simulink model "Duffing_Oszillator_Simulation"  (R2018b)
settings: Solver=VariableStepAuto  StartTime=0.0  StopTime=30  RelTol=1e-3
values from neighbouring files (symbols this model uses):
  a_alpha = 0.95    [Duffing_Oszillator_Parameter.m]
  a_delta = 0.95    [Duffing_Oszillator_Parameter.m]
  alpha_w = 1    [Duffing_Oszillator_Parameter.m]
  beta_w = -1    [Duffing_Oszillator_Parameter.m]
  delta_ksi = (0.3-(-0.3))/(r-1)    (= 0.03)    [Duffing_Oszillator_Parameter.m]
  delta_w = 0.2    [Duffing_Oszillator_Parameter.m]
  eta_alpha = 7*10^(-2)    (= 0.07)    [Duffing_Oszillator_Parameter.m]
  eta_delta = 1.5*10^(-3)    (= 0.0015)    [Duffing_Oszillator_Parameter.m]
  gamma_w = 10    [Duffing_Oszillator_Parameter.m]
  h = 0.001    [Duffing_Oszillator_Parameter.m]
  ksi = linspace(-0.3,0.3,r)    [Duffing_Oszillator_Parameter.m]
  l1 = 10    [Duffing_Oszillator_Parameter.m]
  l2 = 1.75    [Duffing_Oszillator_Parameter.m]
  omega_0 = 6    [Duffing_Oszillator_Parameter.m]
  r = 21    [Duffing_Oszillator_Parameter.m]
  sigma_norm = 0.3    [Duffing_Oszillator_Parameter.m]
undefined symbols (not defined in the file or in its folder): a_theta, DiscIntNeverNeededParam, eta_theta
settings Model: Creator=LENOVO  LastModifiedBy=LENOVO

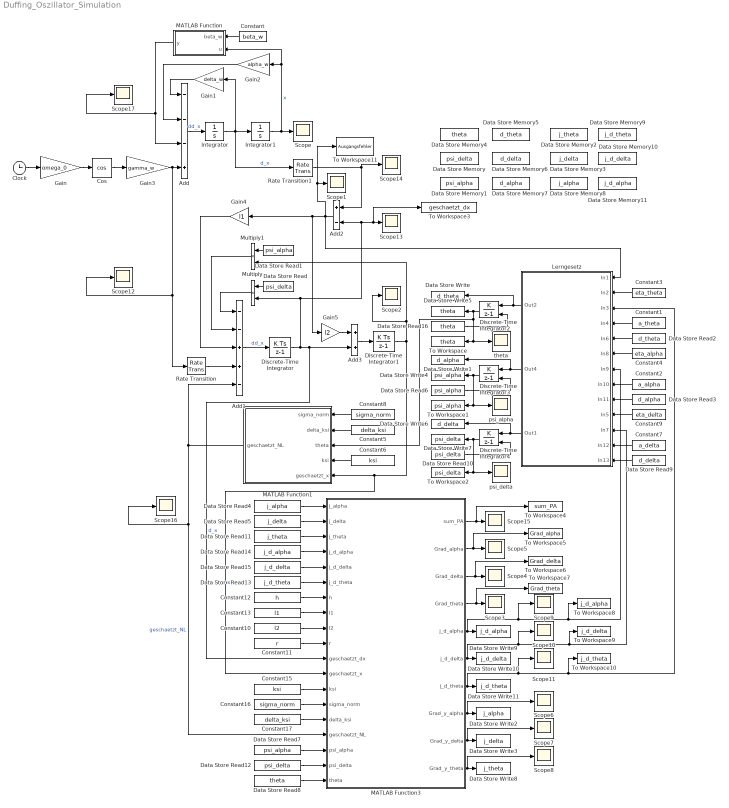
== system Duffing_Oszillator_Simulation ==
  Add : Sum  Inputs=---+
  Add1 : Sum  Inputs=--++-
  Add2 : Sum  Inputs=+-
  Add3 : Sum
  Clock : Clock
  Constant : Constant  Value=beta_w
  Constant1 : Constant  Value=a_theta
  Constant10 : Constant  Value=l2
  Constant11 : Constant  Value=r
  Constant12 : Constant  Value=h
  Constant13 : Constant  Value=l1
  Constant15 : Constant  Value=ksi
  Constant16 : Constant  Value=sigma_norm
  Constant17 : Constant  Value=delta_ksi
  Constant2 : Constant  Value=a_alpha
  Constant3 : Constant  Value=eta_theta
  Constant4 : Constant  Value=eta_alpha
  Constant5 : Constant  Value=delta_ksi
  Constant6 : Constant  Value=ksi
  Constant7 : Constant  Value=a_delta
  Constant8 : Constant  Value=sigma_norm
  Constant9 : Constant  Value=eta_delta
  Cos : Trigonometry  Operator=cos
  Data Store Memory : DataStoreMemory  DataStoreName=psi_delta  ReadBeforeWriteMsg=warning  WriteAfterWriteMsg=warning  WriteAfterReadMsg=warning  InitialValue=0.3  ShowAdditionalParam=off
  Data Store Memory1 : DataStoreMemory  DataStoreName=psi_alpha  ReadBeforeWriteMsg=warning  WriteAfterWriteMsg=warning  WriteAfterReadMsg=warning  InitialValue=1.4  ShowAdditionalParam=off
  Data Store Memory10 : DataStoreMemory  DataStoreName=j_d_delta  ReadBeforeWriteMsg=warning  WriteAfterWriteMsg=warning  WriteAfterReadMsg=warning  ShowAdditionalParam=off
  Data Store Memory11 : DataStoreMemory  DataStoreName=j_d_alpha  ReadBeforeWriteMsg=warning  WriteAfterWriteMsg=warning  WriteAfterReadMsg=warning  ShowAdditionalParam=off
  Data Store Memory2 : DataStoreMemory  DataStoreName=j_theta  ReadBeforeWriteMsg=warning  WriteAfterWriteMsg=warning  WriteAfterReadMsg=warning  InitialValue=zeros(1,r)  ShowAdditionalParam=off
  Data Store Memory3 : DataStoreMemory  DataStoreName=j_delta  ReadBeforeWriteMsg=warning  WriteAfterWriteMsg=warning  WriteAfterReadMsg=warning  ShowAdditionalParam=off
  Data Store Memory4 : DataStoreMemory  DataStoreName=theta  ReadBeforeWriteMsg=warning  WriteAfterWriteMsg=warning  WriteAfterReadMsg=warning  InitialValue=zeros(1,r)  ShowAdditionalParam=off
  Data Store Memory5 : DataStoreMemory  DataStoreName=d_theta  ReadBeforeWriteMsg=warning  WriteAfterWriteMsg=warning  WriteAfterReadMsg=warning  InitialValue=zeros(1,r)  ShowAdditionalParam=off
  Data Store Memory6 : DataStoreMemory  DataStoreName=d_delta  ReadBeforeWriteMsg=warning  WriteAfterWriteMsg=warning  WriteAfterReadMsg=warning  ShowAdditionalParam=off
  Data Store Memory7 : DataStoreMemory  DataStoreName=d_alpha  ReadBeforeWriteMsg=warning  WriteAfterWriteMsg=warning  WriteAfterReadMsg=warning  ShowAdditionalParam=off
  Data Store Memory8 : DataStoreMemory  DataStoreName=j_alpha  ReadBeforeWriteMsg=warning  WriteAfterWriteMsg=warning  WriteAfterReadMsg=warning  ShowAdditionalParam=off
  Data Store Memory9 : DataStoreMemory  DataStoreName=j_d_theta  ReadBeforeWriteMsg=warning  WriteAfterWriteMsg=warning  WriteAfterReadMsg=warning  InitialValue=zeros(1,r)  ShowAdditionalParam=off
  Data Store Read : DataStoreRead  DataStoreName=psi_delta
  Data Store Read1 : DataStoreRead  DataStoreName=psi_alpha
  Data Store Read10 : DataStoreRead  DataStoreName=psi_delta
  Data Store Read11 : DataStoreRead  DataStoreName=j_theta
  Data Store Read12 : DataStoreRead  DataStoreName=psi_delta
  Data Store Read13 : DataStoreRead  DataStoreName=j_d_theta
  Data Store Read14 : DataStoreRead  DataStoreName=j_d_alpha
  Data Store Read15 : DataStoreRead  DataStoreName=j_d_delta
  Data Store Read16 : DataStoreRead  DataStoreName=theta
  Data Store Read2 : DataStoreRead  DataStoreName=d_theta
  Data Store Read3 : DataStoreRead  DataStoreName=d_alpha
  Data Store Read4 : DataStoreRead  DataStoreName=j_alpha
  Data Store Read5 : DataStoreRead  DataStoreName=j_delta
  Data Store Read6 : DataStoreRead  DataStoreName=psi_alpha
  Data Store Read7 : DataStoreRead  DataStoreName=psi_alpha
  Data Store Read8 : DataStoreRead  DataStoreName=theta
  Data Store Read9 : DataStoreRead  DataStoreName=d_delta
  Data Store Write : DataStoreWrite  DataStoreName=d_theta
  Data Store Write1 : DataStoreWrite  DataStoreName=d_alpha
  Data Store Write10 : DataStoreWrite  DataStoreName=j_d_delta
  Data Store Write11 : DataStoreWrite  DataStoreName=j_d_theta
  Data Store Write2 : DataStoreWrite  DataStoreName=j_alpha
  Data Store Write3 : DataStoreWrite  DataStoreName=j_delta
  Data Store Write4 : DataStoreWrite  DataStoreName=psi_alpha
  Data Store Write5 : DataStoreWrite  DataStoreName=theta
  Data Store Write6 : DataStoreWrite  DataStoreName=d_delta
  Data Store Write7 : DataStoreWrite  DataStoreName=psi_delta
  Data Store Write8 : DataStoreWrite  DataStoreName=j_theta
  Data Store Write9 : DataStoreWrite  DataStoreName=j_d_alpha
  Discrete-Time Integrator : DiscreteIntegrator  SampleTime=-1  ICPrevOutput=DiscIntNeverNeededParam  ICPrevScaledInput=DiscIntNeverNeededParam
  Discrete-Time Integrator1 : DiscreteIntegrator  InitialCondition=-0.3  SampleTime=-1  ICPrevOutput=DiscIntNeverNeededParam  ICPrevScaledInput=DiscIntNeverNeededParam
  Discrete-Time Integrator2 : DiscreteIntegrator  IntegratorMethod=Accumulation: Forward Euler  gainval=1  InitialConditionSource=external  SampleTime=-1  ICPrevOutput=DiscIntNeverNeededParam  ICPrevScaledInput=DiscIntNeverNeededParam
  Discrete-Time Integrator3 : DiscreteIntegrator  IntegratorMethod=Accumulation: Forward Euler  gainval=1  InitialConditionSource=external  SampleTime=-1  ICPrevOutput=DiscIntNeverNeededParam  ICPrevScaledInput=DiscIntNeverNeededParam
  Discrete-Time Integrator4 : DiscreteIntegrator  IntegratorMethod=Accumulation: Forward Euler  gainval=1  InitialConditionSource=external  SampleTime=-1  ICPrevOutput=DiscIntNeverNeededParam  ICPrevScaledInput=DiscIntNeverNeededParam
  Gain : Gain  Gain=omega_0
  Gain1 : Gain  Gain=delta_w
  Gain2 : Gain  Gain=alpha_w
  Gain3 : Gain  Gain=gamma_w
  Gain4 : Gain  Gain=l1
  Gain5 : Gain  Gain=l2
  Integrator : Integrator
  Integrator1 : Integrator  InitialCondition=-0.3
  Lerngesetz : Subsystem
  MATLAB Function : MATLAB Function  TreatAsAtomicUnit=on
  MATLAB Function1 : MATLAB Function  TreatAsAtomicUnit=on
  MATLAB Function3 : MATLAB Function  TreatAsAtomicUnit=on
  Multiply : Product
  Multiply1 : Product
  Rate Transition : RateTransition  OutPortSampleTime=0.001
  Rate Transition1 : RateTransition  OutPortSampleTime=0.001
  Scope{,1..17} (18 alike) : Scope
  To Workspace : ToWorkspace  VariableName=theta  SampleTime=-1
      settings: Save2DSignal=2-D array (concatenate along first dimension)
  To Workspace1 : ToWorkspace  VariableName=psi_alpha  SaveFormat=Timeseries  SampleTime=-1
  To Workspace10 : ToWorkspace  VariableName=j_d_theta  SaveFormat=Timeseries  SampleTime=-1
  To Workspace11 : ToWorkspace  VariableName=Ausgangsfehler  SaveFormat=Timeseries  SampleTime=-1
  To Workspace2 : ToWorkspace  VariableName=psi_delta  SaveFormat=Timeseries  SampleTime=-1
  To Workspace3 : ToWorkspace  VariableName=geschaetzt_dx  SampleTime=-1
      settings: Save2DSignal=2-D array (concatenate along first dimension)
  To Workspace4 : ToWorkspace  VariableName=sum_PA  SaveFormat=Timeseries  SampleTime=-1
  To Workspace5 : ToWorkspace  VariableName=Grad_alpha  SaveFormat=Timeseries  SampleTime=-1
  To Workspace6 : ToWorkspace  VariableName=Grad_delta  SaveFormat=Timeseries  SampleTime=-1
  To Workspace7 : ToWorkspace  VariableName=Grad_theta  SaveFormat=Timeseries  SampleTime=-1
  To Workspace8 : ToWorkspace  VariableName=j_d_alpha  SaveFormat=Timeseries  SampleTime=-1
  To Workspace9 : ToWorkspace  VariableName=j_d_delta  SaveFormat=Timeseries  SampleTime=-1
  psi_alpha : Scope
  psi_delta : Scope
  theta : Scope
  wires:
  Clock/1 -> Gain/1
  Gain/1 -> Cos/1
  Cos/1 -> Gain3/1
  Add/1 -> Integrator/1  "dd_x"
  Integrator/1 -> Rate Transition1/1, Gain1/1, Integrator1/1  "d_x"
  Integrator1/1 -> Scope/1, MATLAB Function/2(u), Gain2/1  "x"
  Gain1/1 -> Add/1
  Gain2/1 -> Add/2
  MATLAB Function/1(y) -> Scope17/1, Add/3
  Gain3/1 -> Scope12/1, Rate Transition/1, Add/4
  Constant/1 -> MATLAB Function/1(beta_w)
  Rate Transition/1 -> Add1/4
  Add1/1 -> Discrete-Time Integrator/1  "dd_x"
  Discrete-Time Integrator/1 -> To Workspace3/1, Scope13/1, Add2/2, Multiply/2, Add3/2, MATLAB Function3/11(geschaetzt_dx)  "d_x"
  Rate Transition1/1 -> Add2/1, Scope14/1
  Discrete-Time Integrator1/1 -> MATLAB Function1/5(geschaetzt_x), MATLAB Function3/12(geschaetzt_x), Multiply1/2, Scope2/1  "x"
  Add2/1 -> Scope1/1, To Workspace11/1, Gain4/1, Gain5/1, Lerngesetz/1(In1)
  Multiply/1 -> Add1/1
  Multiply1/1 -> Add1/2
  Data Store Read3/1 -> Lerngesetz/9(In11)
  Constant2/1 -> Lerngesetz/8(In10)
  Data Store Read2/1 -> Lerngesetz/5(In6)
  Data Store Read6/1 -> Discrete-Time Integrator3/2
  Discrete-Time Integrator2/1 -> Data Store Write5/1, theta/1, To Workspace/1, MATLAB Function1/3(theta)
  Constant4/1 -> Lerngesetz/6(In8)
  Constant5/1 -> MATLAB Function1/2(delta_ksi)
  Constant3/1 -> Lerngesetz/2(In2)
  Constant16/1 -> MATLAB Function3/14(sigma_norm)
  Constant12/1 -> MATLAB Function3/7(h)
  Constant8/1 -> MATLAB Function1/1(sigma_norm)
  Constant1/1 -> Lerngesetz/4(In4)
  Discrete-Time Integrator3/1 -> psi_alpha/1, To Workspace1/1, Data Store Write4/1
  Lerngesetz/2(Out4) -> Data Store Write1/1, Discrete-Time Integrator3/1
  Constant17/1 -> MATLAB Function3/15(delta_ksi)
  Constant13/1 -> MATLAB Function3/8(l1)
  MATLAB Function3/8(Grad_y_alpha) -> Scope6/1, Data Store Write2/1
  Constant15/1 -> MATLAB Function3/13(ksi)
  Lerngesetz/1(Out2) -> Discrete-Time Integrator2/1, Data Store Write/1
  MATLAB Function1/1(geschaetzt_NL) -> Add1/5, Scope16/1, MATLAB Function3/16(geschaetzt_NL)  "geschaetzt_NL"
  Constant6/1 -> MATLAB Function1/4(ksi)
  Data Store Read9/1 -> Lerngesetz/13(In13)
  Constant9/1 -> Lerngesetz/10(In5)
  Constant7/1 -> Lerngesetz/12(In12)
  Lerngesetz/3(Out1) -> Discrete-Time Integrator4/1, Data Store Write6/1
  Discrete-Time Integrator4/1 -> psi_delta/1, To Workspace2/1, Data Store Write7/1
  Data Store Read10/1 -> Discrete-Time Integrator4/2
  Data Store Read8/1 -> MATLAB Function3/19(theta)
  MATLAB Function3/9(Grad_y_delta) -> Scope7/1, Data Store Write3/1
  MATLAB Function3/10(Grad_y_theta) -> Scope8/1, Data Store Write8/1
  Data Store Read11/1 -> MATLAB Function3/3(j_theta)
  Constant10/1 -> MATLAB Function3/9(l2)
  Constant11/1 -> MATLAB Function3/10(r)
  Data Store Read13/1 -> MATLAB Function3/6("j_d_theta ")
  MATLAB Function3/7(j_d_theta) -> Scope11/1, Lerngesetz/3(In3), To Workspace10/1, Data Store Write11/1
  MATLAB Function3/6(j_d_delta) -> Scope10/1, Lerngesetz/11(In7), To Workspace9/1, Data Store Write10/1
  MATLAB Function3/5(j_d_alpha) -> Scope9/1, Lerngesetz/7(In9), To Workspace8/1, Data Store Write9/1
  Add3/1 -> Discrete-Time Integrator1/1
  Gain5/1 -> Add3/1
  Gain4/1 -> Add1/3
  Data Store Read15/1 -> MATLAB Function3/5("j_d_delta ")
  Data Store Read14/1 -> MATLAB Function3/4("j_d_alpha ")
  Data Store Read4/1 -> MATLAB Function3/1(j_alpha)
  Data Store Read5/1 -> MATLAB Function3/2(j_delta)
  MATLAB Function3/4(Grad_theta) -> To Workspace7/1, Scope3/1
  MATLAB Function3/3(Grad_delta) -> To Workspace6/1, Scope4/1
  MATLAB Function3/2(Grad_alpha) -> To Workspace5/1, Scope5/1
  MATLAB Function3/1(sum_PA) -> To Workspace4/1, Scope15/1
  Data Store Read16/1 -> Discrete-Time Integrator2/2
  Data Store Read1/1 -> Multiply1/1
  Data Store Read/1 -> Multiply/1
  Data Store Read7/1 -> MATLAB Function3/17(psi_alpha)
  Data Store Read12/1 -> MATLAB Function3/18(psi_delta)

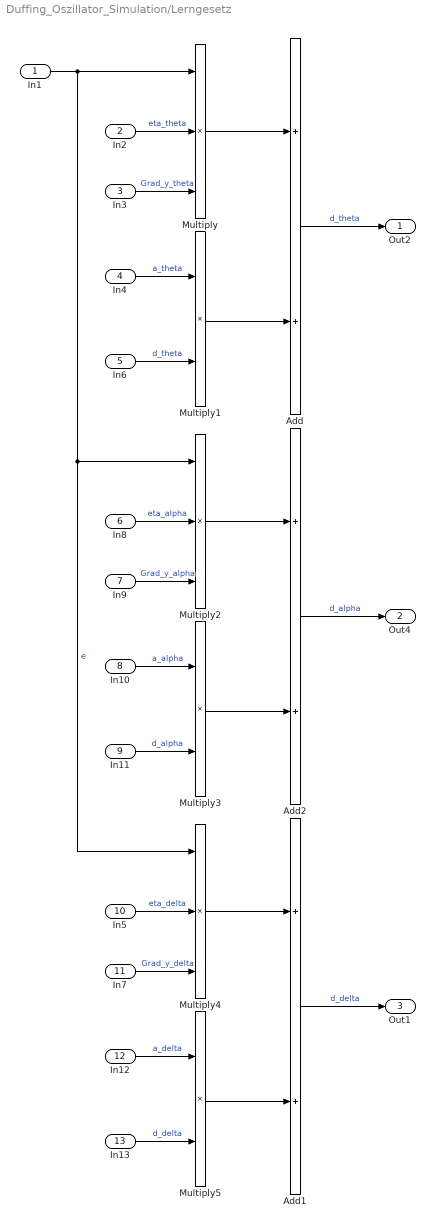
== system Duffing_Oszillator_Simulation/Lerngesetz ==
  In1 : Inport
  In2 : Inport  Port=2
  In3 : Inport  Port=3
  In4 : Inport  Port=4
  In6 : Inport  Port=5
  In8 : Inport  Port=6
  In9 : Inport  Port=7
  In10 : Inport  Port=8
  In11 : Inport  Port=9
  In5 : Inport  Port=10
  In7 : Inport  Port=11
  In12 : Inport  Port=12
  In13 : Inport  Port=13
  Add : Sum  Inputs=2
  Add1 : Sum  Inputs=2
  Add2 : Sum  Inputs=2
  Multiply : Product  Inputs=3
  Multiply1 : Product
  Multiply2 : Product  Inputs=3
  Multiply3 : Product
  Multiply4 : Product  Inputs=3
  Multiply5 : Product
  Out2 : Outport
  Out4 : Outport  Port=2
  Out1 : Outport  Port=3
  wires:
  In3/1 -> Multiply/3  "Grad_y_theta"
  In2/1 -> Multiply/2  "eta_theta"
  In4/1 -> Multiply1/1  "a_theta"
  In6/1 -> Multiply1/2  "d_theta"
  Multiply1/1 -> Add/2
  Multiply/1 -> Add/1
  Add/1 -> Out2/1  "d_theta"
  Add2/1 -> Out4/1  "d_alpha"
  Multiply2/1 -> Add2/1
  Multiply3/1 -> Add2/2
  In11/1 -> Multiply3/2  "d_alpha"
  In10/1 -> Multiply3/1  "a_alpha"
  In8/1 -> Multiply2/2  "eta_alpha"
  In9/1 -> Multiply2/3  "Grad_y_alpha"
  In7/1 -> Multiply4/3  "Grad_y_delta"
  In5/1 -> Multiply4/2  "eta_delta"
  In12/1 -> Multiply5/1  "a_delta"
  In13/1 -> Multiply5/2  "d_delta"
  Multiply5/1 -> Add1/2
  Multiply4/1 -> Add1/1
  Add1/1 -> Out1/1  "d_delta"
  In1/1 -> Multiply/1, Multiply4/1, Multiply2/1  "e"

== matlab function Duffing_Oszillator_Simulation/MATLAB Function ==
  data: beta_w input; u input; y output
function y=NL(beta_w,u)

y=beta_w*u^3;

end

== matlab function Duffing_Oszillator_Simulation/MATLAB Function1 ==
  data: sigma_norm input; delta_ksi input; geschaetzt_NL output; theta input; ksi input; geschaetzt_x input
function geschaetzt_NL=Sum(sigma_norm,delta_ksi,theta,ksi,geschaetzt_x)

Zaehler_AF_GRNN=@(u,ksi) exp(-(u-ksi).^2/(2*sigma_norm^2*delta_ksi^2));
Nenner_AF_GRNN=@(u,ksi) sum(Zaehler_AF_GRNN(u,ksi));
AF_GRNN=@(u,ksi) Zaehler_AF_GRNN(u,ksi)/Nenner_AF_GRNN(u,ksi); %Aktivierungsfunktionen

geschaetzt_NL=sum(theta.*AF_GRNN(geschaetzt_x,ksi));

end

== matlab function Duffing_Oszillator_Simulation/MATLAB Function3 ==
  data: sum_PA output; Grad_alpha output; Grad_delta output; Grad_theta output; j_d_alpha output; j_d_delta output; j_d_theta output; j_alpha input; Grad_y_alpha output; j_delta input; j_theta input; j_d_alpha input; j_d_delta input; j_d_theta input; Grad_y_delta output; h input; l1 input; l2 input; r input; geschaetzt_dx input; geschaetzt_x input; ksi input; sigma_norm input; delta_ksi input; geschaetzt_NL input; psi_alpha input; psi_delta input; theta input; Grad_y_theta output
function [sum_PA,Grad_alpha,Grad_delta,Grad_theta,j_d_alpha,j_d_delta,j_d_theta,Grad_y_alpha,Grad_y_delta,Grad_y_theta]=Partielle_Ableitung(j_alpha,j_delta,j_theta,j_d_alpha,j_d_delta,j_d_theta,h,l1,l2,r,geschaetzt_dx,geschaetzt_x,ksi,sigma_norm,delta_ksi,geschaetzt_NL,psi_alpha,psi_delta,theta)

Zaehler_AF_GRNN=@(u,ksi) exp(-(u-ksi).^2/(2*sigma_norm^2*delta_ksi^2));
Nenner_AF_GRNN=@(u,ksi) sum(Zaehler_AF_GRNN(u,ksi));
AF_GRNN=@(u,ksi) Zaehler_AF_GRNN(u,ksi)/Nenner_AF_GRNN(u,ksi); %Aktivierungsfunktionen

sum_PA=0;

for j=1:r
    sum_PA=sum_PA+Zaehler_AF_GRNN(geschaetzt_x,ksi(j))/Nenner_AF_GRNN(geschaetzt_x,ksi)*(geschaetzt_x-ksi(j))/(sigma_norm^2*delta_ksi^2)*(geschaetzt_NL-theta(j));
end

Grad_alpha=j_alpha*sum_PA;
Grad_delta=j_delta*sum_PA;
Grad_theta=Zaehler_AF_GRNN(geschaetzt_x,ksi)./Nenner_AF_GRNN(geschaetzt_x,ksi)+j_theta.*sum_PA;

f_alpha=-h*Grad_alpha-h*psi_alpha*j_alpha-h*geschaetzt_x;
f_delta=-h*Grad_delta-h*psi_alpha*j_delta-h*geschaetzt_dx;
f_theta=-h.*Grad_theta-h.*psi_alpha.*j_theta;

zwischen_alpha=j_d_alpha;
zwischen_delta=j_d_delta;
zwischen_theta=j_d_theta;

j_d_alpha=(1-h*l1-h*psi_delta)*j_d_alpha+f_alpha;
j_d_delta=(1-h*l1-h*psi_delta)*j_d_delta+f_delta;
j_d_theta=(1-h*l1-h.*psi_delta).*j_d_theta+f_theta;

j_alpha=-h*l2*zwischen_alpha+h*j_d_alpha+j_alpha;
j_delta=-h*l2*zwischen_delta+h*j_d_delta+j_delta;
j_theta=-h*l2.*zwischen_theta+h.*j_d_theta+j_theta;

Grad_y_alpha=j_alpha;
Grad_y_delta=j_delta;
Grad_y_theta=j_theta;
end
